simulink model "Controls"  (R2020a)
settings: Solver=FixedStepDiscrete  StartTime=0.0  StopTime=10  FixedStep=ModelSimTime  RelTol=1e-3
PostLoadFcn:
  | , if any(exist('dsrtsu_mdlpostloadfcn', 'file') == [2, 3, 6]), try dsrtsu_mdlpostloadfcn('Execute', bdroot); catch fprintf('Error in PostLoadFcn (dsrtsu_mdlpostloadfcn) for model "%s":\n %s\n', bdroot, lasterr); end, end,
InitFcn:
  | , if any(exist('rtifpga_mdlclblib', 'file') ~= 0), rtifpga_mdlclblib('Init', bdroot); end,
undefined symbols (not defined in the file): RING_STATUS, TMR
Description:
  | Standard RTI1401 template.
  | Supported MATLAB version:  R2017b.
settings Model: Tag=RTI1401  DSRTSU_INTERNAL_RTI_VER=560  DSRTSU_INTERNAL_RTI_TYPE=rti1401  RTICANMMDATA=struct('GeneralSetupData',struct('modelroot','C:\Users\harjo\Git\MACFormulaGit\MicroAutobox\rings\MFE_Controls','generalsettings',struct('filesettings',struct('destfolder',struct('Name','RTICANMM_FILES','Check',1),'buildfolder',struct('Name','.','Check',1),'AbsDestfolder',struct('Name','C:\Users\harjo\Git\MACFormulaGit\MicroAutobox\rings\MFE_Controls\RTICANMM_FILES'),'AbsBuildfolder',struct('Name','C:\Users\harjo\Git\MACFormulaGit\MicroAutobox\rings\MFE_Controls'))),'options',struct('addpaths',1,'rmpaths',1,'addtrcexclusion',true,'cannavigator',struct('checkmonitoring',0),'show_usrtrc',0,'use_usrtrc',0),'advanced',struct('options',ones(1,100)),'MPSetup',{{}},'RTI',struct('Type','RTI1401','Ver','7.14','Date','02-May-2020'),'modelname','Controls','block','Controls'))  DSRTSU_INTERNAL_RTIFPGA=160  Creator=Harjot  LastModifiedBy=Harjot
settings OptimizationCC: BlockReduction=off  OptimizeBlockIOStorage=off  BufferReuse=off  GlobalBufferReuse=off  ExpressionFolding=off  LocalBlockOutputs=off  OptimizeDataStoreBuffers=off  BusAssignmentInplaceUpdate=off
settings DebuggingCC: ArithmeticOperatorsInVariantConditions=warning
settings HardwareCC: ProdBitPerPointer=32  ProdBitPerSizeT=32  ProdBitPerPtrDiffT=32  ProdLargestAtomicInteger=Integer  ProdEndianess=BigEndian  ProdWordSize=32  ProdHWDeviceType=Custom Processor->Custom  TargetIntDivRoundTo=Zero  TargetEndianess=BigEndian  TargetHWDeviceType=Custom Processor->Custom
settings SFSimCC: SimUseLocalCustomCode=off  MATLABDynamicMemAlloc=off  CustomCodeUndefinedFunction=UseInterfaceOnly
settings RTWCC: Description=dSPACE DS1401 Hardware Platform  SystemTargetFile=rti1401.tlc  MakeCommand=make_rti  TemplateMakefile=rti1401.tmf  RTWUseLocalCustomCode=off
settings CodeAppCC: MaxIdLength=128  StateflowObjectComments=on
settings STFCustomTargetCC: UtilityFuncGeneration=Shared location  ParMdlRefBuildCompliant=on  SystemTargetFile=rti1401.tlc
settings GRTTargetCC: TargetLangStandard=C89/C90 (ANSI)  UtilityFuncGeneration=Shared location  CompOptLevelCompliant=off  ConcurrentExecutionCompliant=off  CombineOutputUpdateFcns=off  MatFileLogging=off  CPPClassGenCompliant=off  UseToolchainInfoCompliant=off
settings ConfigComp: CovMetricSettings=dswe

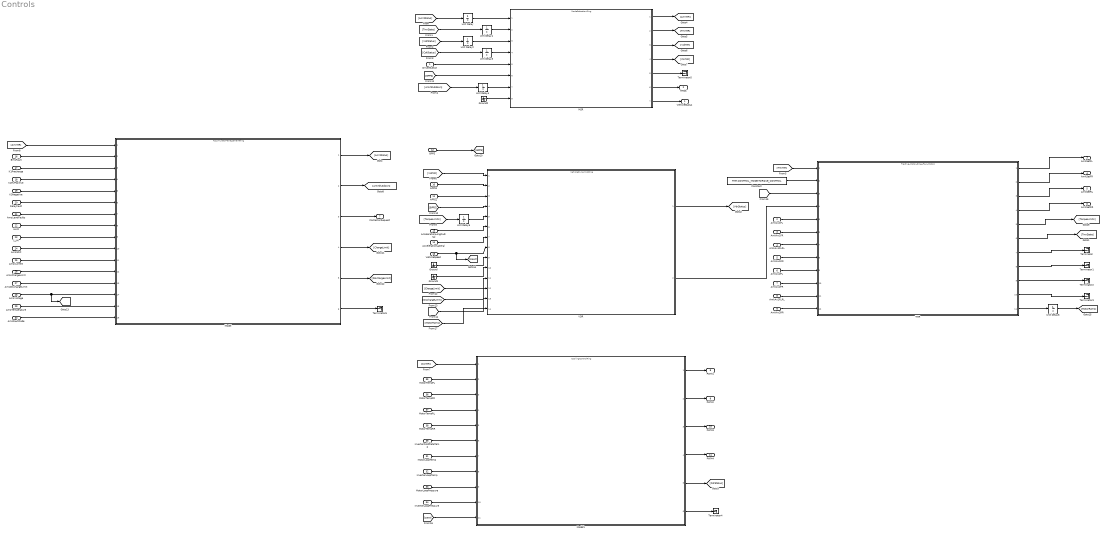
== system Controls ==
  DriverButton : Inport
  AmkAv1FL : Inport  Port=2  OutDataTypeStr=Bus: AmkActualValues1
  AmkAv1FR : Inport  Port=3  OutDataTypeStr=Bus: AmkActualValues1
  AmkAv1FLRL : Inport  Port=4  OutDataTypeStr=Bus: AmkActualValues1
  AmkAv1RR : Inport  Port=5  OutDataTypeStr=Bus: AmkActualValues1
  AmkAv2FL : Inport  Port=6  OutDataTypeStr=Bus: AmkActualValues2
  AmkAv2FR : Inport  Port=7  OutDataTypeStr=Bus: AmkActualValues2
  AmkAv2FLRL : Inport  Port=8  OutDataTypeStr=Bus: AmkActualValues2
  AmkAv2RR : Inport  Port=9  OutDataTypeStr=Bus: AmkActualValues2
  APPS1 : Inport  Port=10  OutDataTypeStr=double
  APPS2 : Inport  Port=11  OutDataTypeStr=double
  BPPS : Inport  Port=12  OutDataTypeStr=double
  AccelerationLongitudinal : Inport  Port=13  OutDataTypeStr=double
  AccelerationLateral : Inport  Port=14  OutDataTypeStr=double
  VehicleSpeed : Inport  Port=15
  BmsFault : Inport  Port=16
  K1Precharge : Inport  Port=17
  K2HvPositive : Inport  Port=18
  K3Negative : Inport  Port=19
  RelayFault : Inport  Port=20
  AmsLevelFaults : Inport  Port=21  OutDataTypeStr=uint8
  HLIM : Inport  Port=22
  LLIM : Inport  Port=23
  AmsSOC : Inport  Port=24
  AmsCurrent : Inport  Port=25
  AmsChargeLimit : Inport  Port=26  OutDataTypeStr=double
  AmsDischargeLimit : Inport  Port=27  OutDataTypeStr=double
  AmsVoltage : Inport  Port=28
  AmsTemperature : Inport  Port=29
  AmsFaultCode : Inport  Port=30  OutDataTypeStr=uint8
  MotorLoopTemp : Inport  Port=31
  InverterLoopTemp : Inport  Port=32
  MotorLoopPressure : Inport  Port=33
  InverterLoopPressure : Inport  Port=34
  MotorTempFL : Inport  Port=35
  MotorTempFR : Inport  Port=36
  MotorTempRL : Inport  Port=37
  MotorTempRR : Inport  Port=38
  InverterColdPlateTemp : Inport  Port=39
  Constant : Constant  Value=TMR.CONTROL_MODE.TORQUE_CONTROL
  Ground : Ground
  Ground1 : Ground
  Ground2 : Ground
  MSR : ModelReference  ModelNameDialog=ModeSelectionRing.slx  SimulationMode=Normal  ModelReferenceVersion=1.232
  Model : ModelReference  ModelNameDialog=AccumulatorManagementRing.slx  SimulationMode=Normal  ModelReferenceVersion=1.70
  Model1 : ModelReference  ModelNameDialog=CoolingControlRing.slx  SimulationMode=Normal  ModelReferenceVersion=1.112
  TMR : ModelReference  ModelNameDialog=Tractive_Motor_Ring_Four_Motors.slx  SimulationMode=Normal  ModelReferenceVersion=1.70
  Terminator{,1..6} (7 alike) : Terminator
  Unit Delay{,1..3} (4 alike) : UnitDelay  InitialCondition=RING_STATUS.OFF  SampleTime=-1  HasFrameUpgradeWarning=on
  Unit Delay4 : UnitDelay  InitialCondition=false  SampleTime=-1  HasFrameUpgradeWarning=on
  Unit Delay5 : UnitDelay  SampleTime=-1  HasFrameUpgradeWarning=on
  Unit Delay6 : UnitDelay  SampleTime=-1  HasFrameUpgradeWarning=on
  VDR : ModelReference  ModelNameDialog=VehicleDynamicsRing.slx  SimulationMode=Normal  ModelReferenceVersion=1.265
  VehicleStatus : Outport  OutDataTypeStr=Enum: VEHICLE_STATUS  VectorParamsAs1DForOutWhenUnconnected=off
  RTDS : Outport  Port=2  VectorParamsAs1DForOutWhenUnconnected=off
  AmkSetFL : Outport  Port=3  OutDataTypeStr=Bus: AmkSetpoints  VectorParamsAs1DForOutWhenUnconnected=off
  AmkSetFR : Outport  Port=4  OutDataTypeStr=Bus: AmkSetpoints  VectorParamsAs1DForOutWhenUnconnected=off
  AmkSetRL : Outport  Port=5  OutDataTypeStr=Bus: AmkSetpoints  VectorParamsAs1DForOutWhenUnconnected=off
  AmkSetRR : Outport  Port=6  OutDataTypeStr=Bus: AmkSetpoints  VectorParamsAs1DForOutWhenUnconnected=off
  ContactorRequest : Outport  Port=7  VectorParamsAs1DForOutWhenUnconnected=off
  PWM1 : Outport  Port=8  VectorParamsAs1DForOutWhenUnconnected=off
  PWM2 : Outport  Port=9  VectorParamsAs1DForOutWhenUnconnected=off
  PWM3 : Outport  Port=10  VectorParamsAs1DForOutWhenUnconnected=off
  PWM4 : Outport  Port=11  VectorParamsAs1DForOutWhenUnconnected=off
  wires:
  Model/1 -> [AmrStatus]
  [AmrStatus] -> Unit Delay/1
  TMR/6 -> [TmrState]
  [TmrState] -> Unit Delay1/1
  VDR/1 -> [VdrStatus]
  [VdrStatus] -> Unit Delay2/1
  Model1/5 -> [CdrStatus]
  [CdrStatus] -> Unit Delay3/1
  DriverButton/1 -> MSR/5
  MSR/1 -> [AmrMR]
  MSR/2 -> [TmrMR]
  MSR/3 -> [VdrMR]
  MSR/4 -> [CcrMR]
  [AmrMR] -> Model/1
  [TmrMR] -> TMR/1
  [VdrMR] -> VDR/1
  [CcrMR] -> Model1/1
  Model/2 -> [AmrShutdown]
  [AmrShutdown] -> Unit Delay4/1
  TMR/7 -> Terminator/1
  TMR/8 -> Terminator1/1
  TMR/9 -> Terminator2/1
  TMR/10 -> Terminator3/1
  TMR/5 -> [TorqueLimits]
  VDR/2 -> TMR/4
  Model1/6 -> Terminator4/1
  AmkAv1FL/1 -> TMR/5
  AmkAv1FR/1 -> TMR/6
  AmkAv1FLRL/1 -> TMR/7
  AmkAv1RR/1 -> TMR/8
  AmkAv2FLRL/1 -> TMR/11
  AmkAv2FL/1 -> TMR/9
  AmkAv2FR/1 -> TMR/10
  AmkAv2RR/1 -> TMR/12
  TMR/1 -> AmkSetFL/1
  TMR/4 -> AmkSetRR/1
  TMR/3 -> AmkSetRL/1
  TMR/2 -> AmkSetFR/1
  Constant/1 -> TMR/2
  APPS1/1 -> VDR/2
  APPS2/1 -> VDR/3
  BPPS/1 -> [BPPS]
  [BPPS] -> VDR/4
  [BPPS] -> MSR/6
  MSR/7 -> VehicleStatus/1
  MSR/6 -> RTDS/1
  MSR/5 -> Terminator5/1
  Ground/1 -> VDR/9
  Ground1/1 -> VDR/10
  AccelerationLateral/1 -> VDR/7
  AccelerationLongitudinal/1 -> VDR/6
  BmsFault/1 -> Model/2
  K1Precharge/1 -> Model/3
  K2HvPositive/1 -> Model/4
  K3Negative/1 -> Model/5
  RelayFault/1 -> Model/6
  AmsLevelFaults/1 -> Model/7
  AmsSOC/1 -> Model/10
  LLIM/1 -> Model/9
  HLIM/1 -> Model/8
  AmsCurrent/1 -> Model/11
  AmsChargeLimit/1 -> Model/12
  AmsDischargeLimit/1 -> Model/13
  AmsVoltage/1 -> [Voltage], Model/14
  AmsTemperature/1 -> Model/15
  AmsFaultCode/1 -> Model/16
  Model/3 -> ContactorRequest/1
  Model/4 -> [ChargeLimit]
  Model/5 -> [DischargeLimit]
  [ChargeLimit] -> VDR/11
  [DischargeLimit] -> VDR/12
  [Voltage] -> VDR/13
  [Voltage] -> TMR/3
  Ground2/1 -> MSR/8
  Model/6 -> Terminator6/1
  MotorLoopTemp/1 -> Model1/7
  InverterLoopTemp/1 -> Model1/8
  MotorLoopPressure/1 -> Model1/9
  InverterLoopPressure/1 -> Model1/10
  [speed] -> Model1/11
  Unit Delay/1 -> MSR/1
  Unit Delay1/1 -> MSR/2
  Unit Delay2/1 -> MSR/3
  Unit Delay3/1 -> MSR/4
  Unit Delay4/1 -> MSR/7
  Unit Delay5/1 -> VDR/5
  MotorTempFL/1 -> Model1/2
  MotorTempFR/1 -> Model1/3
  MotorTempRL/1 -> Model1/4
  MotorTempRR/1 -> Model1/5
  InverterColdPlateTemp/1 -> Model1/6
  VehicleSpeed/1 -> [speed], VDR/8
  [TorqueLimits] -> Unit Delay5/1
  Model1/1 -> PWM1/1
  Model1/2 -> PWM2/1
  Model1/3 -> PWM3/1
  Model1/4 -> PWM4/1
  TMR/11 -> Unit Delay6/1
  [MotorRpms] -> VDR/14
  Unit Delay6/1 -> [MotorRpms]
